simulink model "case4"  (R2024b)
settings: Solver=FixedStepAuto  StartTime=0  StopTime=1  FixedStep=1e-7  RelTol=1e-3
values from neighbouring files (symbols this model uses):
  SG_D_1_D = 0.01056    [IEEE9_case_parameters.m]    (also in case1_parameters.m; case2_parameters.m; case3_parameters.m; case4_parameters.m)
  SG_D_1_EnableSaturation = 0    [IEEE9_case_parameters.m]    (also in case1_parameters.m; case2_parameters.m; case3_parameters.m; case4_parameters.m)
  SG_D_1_f0 = 60    [IEEE9_case_parameters.m]    (also in case1_parameters.m; case2_parameters.m; case3_parameters.m; case4_parameters.m)
  SG_D_1_H = 7.5    [IEEE9_case_parameters.m]    (also in case1_parameters.m; case2_parameters.m; case3_parameters.m; case4_parameters.m)
  SG_D_1_K_A = 20    [IEEE9_case_parameters.m]    (also in case1_parameters.m; case2_parameters.m; case3_parameters.m; case4_parameters.m)
  SG_D_1_K_E = 1.000000e+1    (= 10)    [IEEE9_case_parameters.m]    (also in case1_parameters.m; case2_parameters.m; case3_parameters.m; case4_parameters.m)
  SG_D_1_K_F = 2.363    [IEEE9_case_parameters.m]    (also in case1_parameters.m; case2_parameters.m; case3_parameters.m; case4_parameters.m)
  SG_D_1_K_s = 0.5    [IEEE9_case_parameters.m]    (also in case1_parameters.m = 5; case2_parameters.m = 5; case3_parameters.m = 5; case4_parameters.m = 5)
  SG_D_1_R_a = 0.001088    [IEEE9_case_parameters.m]    (also in case1_parameters.m; case2_parameters.m; case3_parameters.m; case4_parameters.m)
  SG_D_1_S_A = 1    [IEEE9_case_parameters.m]    (also in case1_parameters.m; case2_parameters.m; case3_parameters.m; case4_parameters.m)
  SG_D_1_S_B = 0.103    [IEEE9_case_parameters.m]    (also in case1_parameters.m; case2_parameters.m; case3_parameters.m; case4_parameters.m)
  SG_D_1_S_N = 10.659857    [IEEE9_case_parameters.m]    (also in case1_parameters.m; case2_parameters.m; case3_parameters.m; case4_parameters.m)
  SG_D_1_SpeedPara = 200    [IEEE9_case_parameters.m]    (also in case1_parameters.m; case2_parameters.m; case3_parameters.m; case4_parameters.m)
  SG_D_1_T_0 = 0.720173    [IEEE9_case_parameters.m]    (also in case1_parameters.m = 0.755522; case2_parameters.m = 0.808931; case3_parameters.m = 0.869402; case4_parameters.m = 0.729316)
  SG_D_1_T_1 = 0.3    [IEEE9_case_parameters.m]    (also in case1_parameters.m; case2_parameters.m; case3_parameters.m; case4_parameters.m)
  SG_D_1_T_2 = 0.05    [IEEE9_case_parameters.m]    (also in case1_parameters.m; case2_parameters.m; case3_parameters.m; case4_parameters.m)
  SG_D_1_T_3 = 0.02    [IEEE9_case_parameters.m]    (also in case1_parameters.m; case2_parameters.m; case3_parameters.m; case4_parameters.m)
  SG_D_1_T_4 = 0.005    [IEEE9_case_parameters.m]    (also in case1_parameters.m; case2_parameters.m; case3_parameters.m; case4_parameters.m)
  SG_D_1_T_A = 0.02    [IEEE9_case_parameters.m]    (also in case1_parameters.m; case2_parameters.m; case3_parameters.m; case4_parameters.m)
  SG_D_1_T_dd = 8.000000e+0    (= 8)    [IEEE9_case_parameters.m]    (also in case1_parameters.m; case2_parameters.m; case3_parameters.m; case4_parameters.m)
  SG_D_1_T_ddd = 0.04    [IEEE9_case_parameters.m]    (also in case1_parameters.m; case2_parameters.m; case3_parameters.m; case4_parameters.m)
  SG_D_1_T_E = 0.314    [IEEE9_case_parameters.m]    (also in case1_parameters.m; case2_parameters.m; case3_parameters.m; case4_parameters.m)
  SG_D_1_T_F = 0.35    [IEEE9_case_parameters.m]    (also in case1_parameters.m; case2_parameters.m; case3_parameters.m; case4_parameters.m)
  SG_D_1_T_qd = 0.8    [IEEE9_case_parameters.m]    (also in case1_parameters.m; case2_parameters.m; case3_parameters.m; case4_parameters.m)
  SG_D_1_T_qdd = 0.02    [IEEE9_case_parameters.m]    (also in case1_parameters.m; case2_parameters.m; case3_parameters.m; case4_parameters.m)
  SG_D_1_T_speed = 0.1    [IEEE9_case_parameters.m]    (also in case1_parameters.m = 200; case2_parameters.m = 200; case3_parameters.m = 200; case4_parameters.m = 200)
  SG_D_1_T_w = 0.5    [IEEE9_case_parameters.m]    (also in case1_parameters.m; case2_parameters.m; case3_parameters.m; case4_parameters.m)
  SG_D_1_V_ref = 1.990276    [IEEE9_case_parameters.m]    (also in case1_parameters.m = 2.042296; case2_parameters.m = 2.051388; case3_parameters.m = 2.089584; case4_parameters.m = 2.01845)
  SG_D_1_w_ref = 376.991118    [IEEE9_case_parameters.m]    (also in case1_parameters.m; case2_parameters.m; case3_parameters.m; case4_parameters.m)
  SG_D_1_wb = 6.000000e+1    (= 60)    [IEEE9_case_parameters.m]    (also in case1_parameters.m; case2_parameters.m; case3_parameters.m; case4_parameters.m)
  SG_D_1_x_d = 1.9    [IEEE9_case_parameters.m]    (also in case1_parameters.m; case2_parameters.m; case3_parameters.m; case4_parameters.m)
  SG_D_1_x_dd = 0.302    [IEEE9_case_parameters.m]    (also in case1_parameters.m; case2_parameters.m; case3_parameters.m; case4_parameters.m)
  SG_D_1_x_ddd = 0.204    [IEEE9_case_parameters.m]    (also in case1_parameters.m; case2_parameters.m; case3_parameters.m; case4_parameters.m)
  SG_D_1_x_l = 0.05    [IEEE9_case_parameters.m]    (also in case1_parameters.m; case2_parameters.m; case3_parameters.m; case4_parameters.m)
  SG_D_1_x_q = 1.3    [IEEE9_case_parameters.m]    (also in case1_parameters.m; case2_parameters.m; case3_parameters.m; case4_parameters.m)
  SG_D_1_x_qd = 0.5    [IEEE9_case_parameters.m]    (also in case1_parameters.m; case2_parameters.m; case3_parameters.m; case4_parameters.m)
  SG_D_1_x_qdd = 0.3    [IEEE9_case_parameters.m]    (also in case1_parameters.m; case2_parameters.m; case3_parameters.m; case4_parameters.m)
  SG_D_2_D = 0.02    [IEEE9_case_parameters.m]    (also in case1_parameters.m; case2_parameters.m; case3_parameters.m; case4_parameters.m)
  SG_D_2_EnableSaturation = 0    [IEEE9_case_parameters.m]    (also in case1_parameters.m; case2_parameters.m; case3_parameters.m; case4_parameters.m)
  SG_D_2_f0 = 60    [IEEE9_case_parameters.m]    (also in case1_parameters.m; case2_parameters.m; case3_parameters.m; case4_parameters.m)
  SG_D_2_H = 8.000000e+0    (= 8)    [IEEE9_case_parameters.m]    (also in case1_parameters.m; case2_parameters.m; case3_parameters.m; case4_parameters.m)
  SG_D_2_K_A = 20    [IEEE9_case_parameters.m]    (also in case1_parameters.m; case2_parameters.m; case3_parameters.m; case4_parameters.m)
  SG_D_2_K_E = 1.000000e+1    (= 10)    [IEEE9_case_parameters.m]    (also in case1_parameters.m; case2_parameters.m; case3_parameters.m; case4_parameters.m)
  SG_D_2_K_F = 2.363    [IEEE9_case_parameters.m]    (also in case1_parameters.m; case2_parameters.m; case3_parameters.m; case4_parameters.m)
  SG_D_2_K_s = 0.5    [IEEE9_case_parameters.m]    (also in case1_parameters.m = 4; case2_parameters.m = 4; case3_parameters.m = 4; case4_parameters.m = 4)
  SG_D_2_R_a = 0.001088    [IEEE9_case_parameters.m]    (also in case1_parameters.m; case2_parameters.m; case3_parameters.m; case4_parameters.m)
  SG_D_2_S_A = 1    [IEEE9_case_parameters.m]    (also in case1_parameters.m; case2_parameters.m; case3_parameters.m; case4_parameters.m)
  SG_D_2_S_B = 0.103    [IEEE9_case_parameters.m]    (also in case1_parameters.m; case2_parameters.m; case3_parameters.m; case4_parameters.m)
  SG_D_2_S_N = 10.659857    [IEEE9_case_parameters.m]    (also in case1_parameters.m; case2_parameters.m; case3_parameters.m; case4_parameters.m)
  SG_D_2_SpeedPara = 200    [IEEE9_case_parameters.m]    (also in case1_parameters.m; case2_parameters.m; case3_parameters.m; case4_parameters.m)
  SG_D_2_T_0 = 1.632913    [IEEE9_case_parameters.m]    (also in case1_parameters.m = 1.632925; case2_parameters.m = 1.632915; case3_parameters.m = 1.632914; case4_parameters.m = 1.632927)
  SG_D_2_T_1 = 0.2    [IEEE9_case_parameters.m]    (also in case1_parameters.m; case2_parameters.m; case3_parameters.m; case4_parameters.m)
  SG_D_2_T_2 = 0.05    [IEEE9_case_parameters.m]    (also in case1_parameters.m; case2_parameters.m; case3_parameters.m; case4_parameters.m)
  SG_D_2_T_3 = 0.02    [IEEE9_case_parameters.m]    (also in case1_parameters.m; case2_parameters.m; case3_parameters.m; case4_parameters.m)
  SG_D_2_T_4 = 0.005    [IEEE9_case_parameters.m]    (also in case1_parameters.m; case2_parameters.m; case3_parameters.m; case4_parameters.m)
  SG_D_2_T_A = 0.02    [IEEE9_case_parameters.m]    (also in case1_parameters.m; case2_parameters.m; case3_parameters.m; case4_parameters.m)
  SG_D_2_T_dd = 7.9    [IEEE9_case_parameters.m]    (also in case1_parameters.m; case2_parameters.m; case3_parameters.m; case4_parameters.m)
  SG_D_2_T_ddd = 0.04    [IEEE9_case_parameters.m]    (also in case1_parameters.m; case2_parameters.m; case3_parameters.m; case4_parameters.m)
  SG_D_2_T_E = 0.314    [IEEE9_case_parameters.m]    (also in case1_parameters.m; case2_parameters.m; case3_parameters.m; case4_parameters.m)
  SG_D_2_T_F = 0.35    [IEEE9_case_parameters.m]    (also in case1_parameters.m; case2_parameters.m; case3_parameters.m; case4_parameters.m)
  SG_D_2_T_qd = 0.8    [IEEE9_case_parameters.m]    (also in case1_parameters.m; case2_parameters.m; case3_parameters.m; case4_parameters.m)
  SG_D_2_T_qdd = 0.015    [IEEE9_case_parameters.m]    (also in case1_parameters.m; case2_parameters.m; case3_parameters.m; case4_parameters.m)
  SG_D_2_T_speed = 0.1    [IEEE9_case_parameters.m]    (also in case1_parameters.m = 150; case2_parameters.m = 150; case3_parameters.m = 150; case4_parameters.m = 150)
  SG_D_2_T_w = 0.35    [IEEE9_case_parameters.m]    (also in case1_parameters.m; case2_parameters.m; case3_parameters.m; case4_parameters.m)
  SG_D_2_V_ref = 2.58547    [IEEE9_case_parameters.m]    (also in case1_parameters.m = 2.597896; case2_parameters.m = 2.587136; case3_parameters.m = 2.586042; case4_parameters.m = 2.599679)
  SG_D_2_w_ref = 376.991118    [IEEE9_case_parameters.m]    (also in case1_parameters.m; case2_parameters.m; case3_parameters.m; case4_parameters.m)
  SG_D_2_wb = 6.000000e+1    (= 60)    [IEEE9_case_parameters.m]    (also in case1_parameters.m; case2_parameters.m; case3_parameters.m; case4_parameters.m)
  SG_D_2_x_d = 1.8    [IEEE9_case_parameters.m]    (also in case1_parameters.m; case2_parameters.m; case3_parameters.m; case4_parameters.m)
  SG_D_2_x_dd = 0.302    [IEEE9_case_parameters.m]    (also in case1_parameters.m; case2_parameters.m; case3_parameters.m; case4_parameters.m)
  SG_D_2_x_ddd = 0.204    [IEEE9_case_parameters.m]    (also in case1_parameters.m; case2_parameters.m; case3_parameters.m; case4_parameters.m)
  SG_D_2_x_l = 0.05    [IEEE9_case_parameters.m]    (also in case1_parameters.m; case2_parameters.m; case3_parameters.m; case4_parameters.m)
  SG_D_2_x_q = 1.25    [IEEE9_case_parameters.m]    (also in case1_parameters.m; case2_parameters.m; case3_parameters.m; case4_parameters.m)
  SG_D_2_x_qd = 0.5    [IEEE9_case_parameters.m]    (also in case1_parameters.m; case2_parameters.m; case3_parameters.m; case4_parameters.m)
  SG_D_2_x_qdd = 0.3    [IEEE9_case_parameters.m]    (also in case1_parameters.m; case2_parameters.m; case3_parameters.m; case4_parameters.m)
  SG_D_3_D = 0.02    [IEEE9_case_parameters.m]    (also in case1_parameters.m; case2_parameters.m; case3_parameters.m; case4_parameters.m)
  SG_D_3_EnableSaturation = 0    [IEEE9_case_parameters.m]    (also in case1_parameters.m; case2_parameters.m; case3_parameters.m; case4_parameters.m)
  SG_D_3_f0 = 60    [IEEE9_case_parameters.m]    (also in case1_parameters.m; case2_parameters.m; case3_parameters.m; case4_parameters.m)
  SG_D_3_H = 7.7    [IEEE9_case_parameters.m]    (also in case1_parameters.m; case2_parameters.m; case3_parameters.m; case4_parameters.m)
  SG_D_3_K_A = 20    [IEEE9_case_parameters.m]    (also in case1_parameters.m; case2_parameters.m; case3_parameters.m; case4_parameters.m)
  SG_D_3_K_E = 1.000000e+1    (= 10)    [IEEE9_case_parameters.m]    (also in case1_parameters.m; case2_parameters.m; case3_parameters.m; case4_parameters.m)
  SG_D_3_K_F = 2.363    [IEEE9_case_parameters.m]    (also in case1_parameters.m; case2_parameters.m; case3_parameters.m; case4_parameters.m)
  SG_D_3_K_s = 0.2    [IEEE9_case_parameters.m]    (also in case1_parameters.m = 2; case2_parameters.m = 2; case3_parameters.m = 2; case4_parameters.m = 2)
  SG_D_3_R_a = 0.001088    [IEEE9_case_parameters.m]    (also in case1_parameters.m; case2_parameters.m; case3_parameters.m; case4_parameters.m)
  SG_D_3_S_A = 1    [IEEE9_case_parameters.m]    (also in case1_parameters.m; case2_parameters.m; case3_parameters.m; case4_parameters.m)
  SG_D_3_S_B = 0.103    [IEEE9_case_parameters.m]    (also in case1_parameters.m; case2_parameters.m; case3_parameters.m; case4_parameters.m)
  SG_D_3_S_N = 10.659857    [IEEE9_case_parameters.m]    (also in case1_parameters.m; case2_parameters.m; case3_parameters.m; case4_parameters.m)
  SG_D_3_SpeedPara = 200    [IEEE9_case_parameters.m]    (also in case1_parameters.m; case2_parameters.m; case3_parameters.m; case4_parameters.m)
  SG_D_3_T_0 = 0.850788    [IEEE9_case_parameters.m]    (also in case1_parameters.m = 0.850786; case2_parameters.m = 0.850787; case3_parameters.m; case4_parameters.m = 0.850786)
  SG_D_3_T_1 = 0.2    [IEEE9_case_parameters.m]    (also in case1_parameters.m; case2_parameters.m; case3_parameters.m; case4_parameters.m)
  SG_D_3_T_2 = 0.05    [IEEE9_case_parameters.m]    (also in case1_parameters.m; case2_parameters.m; case3_parameters.m; case4_parameters.m)
  SG_D_3_T_3 = 0.02    [IEEE9_case_parameters.m]    (also in case1_parameters.m; case2_parameters.m; case3_parameters.m; case4_parameters.m)
  SG_D_3_T_4 = 0.005    [IEEE9_case_parameters.m]    (also in case1_parameters.m; case2_parameters.m; case3_parameters.m; case4_parameters.m)
  SG_D_3_T_A = 0.02    [IEEE9_case_parameters.m]    (also in case1_parameters.m; case2_parameters.m; case3_parameters.m; case4_parameters.m)
  SG_D_3_T_dd = 8.1    [IEEE9_case_parameters.m]    (also in case1_parameters.m; case2_parameters.m; case3_parameters.m; case4_parameters.m)
  SG_D_3_T_ddd = 0.04    [IEEE9_case_parameters.m]    (also in case1_parameters.m; case2_parameters.m; case3_parameters.m; case4_parameters.m)
  SG_D_3_T_E = 0.314    [IEEE9_case_parameters.m]    (also in case1_parameters.m; case2_parameters.m; case3_parameters.m; case4_parameters.m)
  SG_D_3_T_F = 0.35    [IEEE9_case_parameters.m]    (also in case1_parameters.m; case2_parameters.m; case3_parameters.m; case4_parameters.m)
  SG_D_3_T_qd = 0.8    [IEEE9_case_parameters.m]    (also in case1_parameters.m; case2_parameters.m; case3_parameters.m; case4_parameters.m)
  SG_D_3_T_qdd = 0.015    [IEEE9_case_parameters.m]    (also in case1_parameters.m; case2_parameters.m; case3_parameters.m; case4_parameters.m)
  SG_D_3_T_speed = 0.1    [IEEE9_case_parameters.m]    (also in case1_parameters.m = 180; case2_parameters.m = 180; case3_parameters.m = 180; case4_parameters.m = 180)
  SG_D_3_T_w = 0.4    [IEEE9_case_parameters.m]    (also in case1_parameters.m; case2_parameters.m; case3_parameters.m; case4_parameters.m)
  SG_D_3_V_ref = 1.892727    [IEEE9_case_parameters.m]    (also in case1_parameters.m = 1.906439; case2_parameters.m = 1.895535; case3_parameters.m = 1.892105; case4_parameters.m = 1.906598)
  SG_D_3_w_ref = 376.991118    [IEEE9_case_parameters.m]    (also in case1_parameters.m; case2_parameters.m; case3_parameters.m; case4_parameters.m)
  SG_D_3_wb = 6.000000e+1    (= 60)    [IEEE9_case_parameters.m]    (also in case1_parameters.m; case2_parameters.m; case3_parameters.m; case4_parameters.m)
  SG_D_3_x_d = 1.85    [IEEE9_case_parameters.m]    (also in case1_parameters.m; case2_parameters.m; case3_parameters.m; case4_parameters.m)
  SG_D_3_x_dd = 0.302    [IEEE9_case_parameters.m]    (also in case1_parameters.m; case2_parameters.m; case3_parameters.m; case4_parameters.m)
  SG_D_3_x_ddd = 0.204    [IEEE9_case_parameters.m]    (also in case1_parameters.m; case2_parameters.m; case3_parameters.m; case4_parameters.m)
  SG_D_3_x_l = 0.05    [IEEE9_case_parameters.m]    (also in case1_parameters.m; case2_parameters.m; case3_parameters.m; case4_parameters.m)
  SG_D_3_x_q = 1.2    [IEEE9_case_parameters.m]    (also in case1_parameters.m; case2_parameters.m; case3_parameters.m; case4_parameters.m)
  SG_D_3_x_qd = 0.5    [IEEE9_case_parameters.m]    (also in case1_parameters.m; case2_parameters.m; case3_parameters.m; case4_parameters.m)
  SG_D_3_x_qdd = 0.3    [IEEE9_case_parameters.m]    (also in case1_parameters.m; case2_parameters.m; case3_parameters.m; case4_parameters.m)
(part 4 of 12)

== system case4/AC_1/d_vq_bus_7_block ==
  note: d_vq_bus_7 in case4
      | $2106.09563369148\,\mathrm{iq}_{\mathrm{bus},7}-376.991118430775\,\mathrm{vd}_{\mathrm{bus},7}$
      | Automatically generated on 2025-10-31 19:07:32 .
  Alge_iq_bus_7_a187d : Inport
  State_vd_bus_7_abf75 : Inport  Port=2
  Constant_2106.09563369148_e620c : Constant  Value=2106.09563369148
  Constant_376.991118430775_7228e : Constant  Value=376.991118430775
  Product_2f562 : Product
  Product_863a6 : Product
  Subtract_ba788 : Sum  Inputs=+-
  Blockout_d_vq_bus_7_f8968 : Outport
  wires:
  Constant_2106.09563369148_e620c/1 -> Product_2f562/1
  Product_863a6/1 -> Subtract_ba788/2
  Alge_iq_bus_7_a187d/1 -> Product_2f562/2
  Constant_376.991118430775_7228e/1 -> Product_863a6/1
  Subtract_ba788/1 -> Blockout_d_vq_bus_7_f8968/1
  State_vd_bus_7_abf75/1 -> Product_863a6/2
  Product_2f562/1 -> Subtract_ba788/1

== system case4/AC_1/d_vq_bus_8_block ==
  note: d_vq_bus_8 in case4
      | $1657.10381727813\,\mathrm{iq}_{\mathrm{bus},8}-376.991118430775\,\mathrm{vd}_{\mathrm{bus},8}$
      | Automatically generated on 2025-10-31 19:07:34 .
  Alge_iq_bus_8_9b29c : Inport
  State_vd_bus_8_14918 : Inport  Port=2
  Constant_1657.10381727813_3cf0f : Constant  Value=1657.10381727813
  Constant_376.991118430775_38ca6 : Constant  Value=376.991118430775
  Product_3ddfe : Product
  Product_639f3 : Product
  Subtract_26c78 : Sum  Inputs=+-
  Blockout_d_vq_bus_8_3ee0b : Outport
  wires:
  Constant_1657.10381727813_3cf0f/1 -> Product_3ddfe/1
  Constant_376.991118430775_38ca6/1 -> Product_639f3/1
  Alge_iq_bus_8_9b29c/1 -> Product_3ddfe/2
  State_vd_bus_8_14918/1 -> Product_639f3/2
  Product_3ddfe/1 -> Subtract_26c78/1
  Product_639f3/1 -> Subtract_26c78/2
  Subtract_26c78/1 -> Blockout_d_vq_bus_8_3ee0b/1

== system case4/AC_1/d_vq_bus_9_block ==
  note: d_vq_bus_9 in case4
      | $1564.27849971276\,\mathrm{iq}_{\mathrm{bus},9}-376.991118430775\,\mathrm{vd}_{\mathrm{bus},9}$
      | Automatically generated on 2025-10-31 19:07:35 .
  Alge_iq_bus_9_c8820 : Inport
  State_vd_bus_9_5e7c3 : Inport  Port=2
  Constant_1564.27849971276_69eb4 : Constant  Value=1564.27849971276
  Constant_376.991118430775_a1ef0 : Constant  Value=376.991118430775
  Product_adb94 : Product
  Product_c35c3 : Product
  Subtract_0c4fa : Sum  Inputs=+-
  Blockout_d_vq_bus_9_ae447 : Outport
  wires:
  Constant_1564.27849971276_69eb4/1 -> Product_c35c3/1
  Constant_376.991118430775_a1ef0/1 -> Product_adb94/1
  Alge_iq_bus_9_c8820/1 -> Product_c35c3/2
  State_vd_bus_9_5e7c3/1 -> Product_adb94/2
  Product_c35c3/1 -> Subtract_0c4fa/1
  Product_adb94/1 -> Subtract_0c4fa/2
  Subtract_0c4fa/1 -> Blockout_d_vq_bus_9_ae447/1

== system case4/AC_1/id_bus_1_block ==
  note: id_bus_1 in case4
      | $\mathrm{id}_{\mathrm{SG},D,1}-\mathrm{id}_{\mathrm{line},1,4}$
      | Automatically generated on 2025-10-31 19:08:04 .
  Input_id_SG_D_1_73334 : Inport
  State_id_line_1_4_ee531 : Inport  Port=2
  Subtract_490f2 : Sum  Inputs=+-
  Blockout_id_bus_1_00a24 : Outport
  wires:
  Input_id_SG_D_1_73334/1 -> Subtract_490f2/1
  State_id_line_1_4_ee531/1 -> Subtract_490f2/2
  Subtract_490f2/1 -> Blockout_id_bus_1_00a24/1

== system case4/AC_1/id_bus_2_block ==
  note: id_bus_2 in case4
      | $\mathrm{id}_{\mathrm{SG},D,2}+\mathrm{id}_{\mathrm{line},8,2}$
      | Automatically generated on 2025-10-31 19:08:07 .
  Input_id_SG_D_2_fbcda : Inport
  State_id_line_8_2_cfe5e : Inport  Port=2
  Add_11ac2 : Sum
  Blockout_id_bus_2_d0074 : Outport
  wires:
  Input_id_SG_D_2_fbcda/1 -> Add_11ac2/1
  State_id_line_8_2_cfe5e/1 -> Add_11ac2/2
  Add_11ac2/1 -> Blockout_id_bus_2_d0074/1

== system case4/AC_1/id_bus_3_block ==
  note: id_bus_3 in case4
      | $\mathrm{id}_{\mathrm{SG},D,3}-\mathrm{id}_{\mathrm{line},3,6}$
      | Automatically generated on 2025-10-31 19:08:09 .
  Input_id_SG_D_3_1ed07 : Inport
  State_id_line_3_6_05496 : Inport  Port=2
  Subtract_1ce5f : Sum  Inputs=+-
  Blockout_id_bus_3_9729d : Outport
  wires:
  Input_id_SG_D_3_1ed07/1 -> Subtract_1ce5f/1
  State_id_line_3_6_05496/1 -> Subtract_1ce5f/2
  Subtract_1ce5f/1 -> Blockout_id_bus_3_9729d/1

== system case4/AC_1/id_bus_4_block ==
  note: id_bus_4 in case4
      | $\mathrm{id}_{\mathrm{line},1,4}-\mathrm{id}_{\mathrm{line},4,5}+\mathrm{id}_{\mathrm{line},9,4}$
      | Automatically generated on 2025-10-31 19:08:10 .
  State_id_line_1_4_a86fb : Inport
  State_id_line_4_5_25293 : Inport  Port=2
  State_id_line_9_4_32915 : Inport  Port=3
  Add_ea890 : Sum
  Subtract_f741b : Sum  Inputs=+-
  Blockout_id_bus_4_42f24 : Outport
  wires:
  State_id_line_9_4_32915/1 -> Add_ea890/2
  State_id_line_1_4_a86fb/1 -> Subtract_f741b/1
  State_id_line_4_5_25293/1 -> Subtract_f741b/2
  Subtract_f741b/1 -> Add_ea890/1
  Add_ea890/1 -> Blockout_id_bus_4_42f24/1

== system case4/AC_1/id_bus_5_block ==
  note: id_bus_5 in case4
      | $\mathrm{id}_{\mathrm{line},4,5}-\mathrm{id}_{\mathrm{load},5}-\mathrm{id}_{\mathrm{line},5,6}$
      | Automatically generated on 2025-10-31 19:08:12 .
  State_id_load_5_ce210 : Inport
  State_id_line_4_5_86da7 : Inport  Port=2
  State_id_line_5_6_37460 : Inport  Port=3
  Add_495f7 : Sum
  Constant_-1_405b2 : Constant  Value=-1
  Product_41ded : Product
  Subtract_56e37 : Sum  Inputs=+-
  Blockout_id_bus_5_00d6f : Outport
  wires:
  Subtract_56e37/1 -> Blockout_id_bus_5_00d6f/1
  State_id_line_4_5_86da7/1 -> Add_495f7/2
  Constant_-1_405b2/1 -> Product_41ded/1
  Add_495f7/1 -> Subtract_56e37/1
  State_id_load_5_ce210/1 -> Product_41ded/2
  Product_41ded/1 -> Add_495f7/1
  State_id_line_5_6_37460/1 -> Subtract_56e37/2

== system case4/AC_1/id_bus_6_block ==
  note: id_bus_6 in case4
      | $\mathrm{id}_{\mathrm{line},3,6}+\mathrm{id}_{\mathrm{line},5,6}-\mathrm{id}_{\mathrm{line},6,7}$
      | Automatically generated on 2025-10-31 19:08:13 .
  State_id_line_3_6_de78e : Inport
  State_id_line_5_6_1a694 : Inport  Port=2
  State_id_line_6_7_1ddf3 : Inport  Port=3
  Add_b3029 : Sum
  Subtract_06215 : Sum  Inputs=+-
  Blockout_id_bus_6_23bdb : Outport
  wires:
  State_id_line_6_7_1ddf3/1 -> Subtract_06215/2
  State_id_line_3_6_de78e/1 -> Add_b3029/1
  State_id_line_5_6_1a694/1 -> Add_b3029/2
  Add_b3029/1 -> Subtract_06215/1
  Subtract_06215/1 -> Blockout_id_bus_6_23bdb/1

== system case4/AC_1/id_bus_7_block ==
  note: id_bus_7 in case4
      | $\mathrm{id}_{\mathrm{line},6,7}-\mathrm{id}_{\mathrm{load},7}-\mathrm{id}_{\mathrm{line},7,8}$
      | Automatically generated on 2025-10-31 19:08:14 .
  State_id_load_7_08a11 : Inport
  State_id_line_6_7_3a993 : Inport  Port=2
  State_id_line_7_8_7bb7d : Inport  Port=3
  Add_165c5 : Sum
  Constant_-1_3b2a9 : Constant  Value=-1
  Product_6f470 : Product
  Subtract_6c348 : Sum  Inputs=+-
  Blockout_id_bus_7_de2dd : Outport
  wires:
  Subtract_6c348/1 -> Blockout_id_bus_7_de2dd/1
  State_id_line_6_7_3a993/1 -> Add_165c5/2
  Constant_-1_3b2a9/1 -> Product_6f470/1
  Add_165c5/1 -> Subtract_6c348/1
  State_id_load_7_08a11/1 -> Product_6f470/2
  Product_6f470/1 -> Add_165c5/1
  State_id_line_7_8_7bb7d/1 -> Subtract_6c348/2

== system case4/AC_1/id_bus_8_block ==
  note: id_bus_8 in case4
      | $\mathrm{id}_{\mathrm{line},7,8}-\mathrm{id}_{\mathrm{line},8,2}-\mathrm{id}_{\mathrm{line},8,9}$
      | Automatically generated on 2025-10-31 19:08:16 .
  State_id_line_7_8_b4fab : Inport
  State_id_line_8_2_e242b : Inport  Port=2
  State_id_line_8_9_3adb9 : Inport  Port=3
  Subtract_0bae2 : Sum  Inputs=+-
  Subtract_32f21 : Sum  Inputs=+-
  Blockout_id_bus_8_7113f : Outport
  wires:
  State_id_line_8_9_3adb9/1 -> Subtract_32f21/2
  State_id_line_7_8_b4fab/1 -> Subtract_0bae2/1
  State_id_line_8_2_e242b/1 -> Subtract_0bae2/2
  Subtract_0bae2/1 -> Subtract_32f21/1
  Subtract_32f21/1 -> Blockout_id_bus_8_7113f/1

== system case4/AC_1/id_bus_9_block ==
  note: id_bus_9 in case4
      | $\mathrm{id}_{\mathrm{line},8,9}-\mathrm{id}_{\mathrm{load},9}-\mathrm{id}_{\mathrm{line},9,4}$
      | Automatically generated on 2025-10-31 19:08:17 .
  State_id_load_9_f6d0c : Inport
  State_id_line_8_9_502b6 : Inport  Port=2
  State_id_line_9_4_0d307 : Inport  Port=3
  Add_18cdf : Sum
  Constant_-1_14996 : Constant  Value=-1
  Product_22f20 : Product
  Subtract_385ae : Sum  Inputs=+-
  Blockout_id_bus_9_09ef3 : Outport
  wires:
  Subtract_385ae/1 -> Blockout_id_bus_9_09ef3/1
  State_id_line_8_9_502b6/1 -> Add_18cdf/2
  Constant_-1_14996/1 -> Product_22f20/1
  Add_18cdf/1 -> Subtract_385ae/1
  State_id_load_9_f6d0c/1 -> Product_22f20/2
  Product_22f20/1 -> Add_18cdf/1
  State_id_line_9_4_0d307/1 -> Subtract_385ae/2

== system case4/AC_1/iq_bus_1_block ==
  note: iq_bus_1 in case4
      | $\mathrm{iq}_{\mathrm{SG},D,1}-\mathrm{iq}_{\mathrm{line},1,4}$
      | Automatically generated on 2025-10-31 19:08:05 .
  Input_iq_SG_D_1_3d98d : Inport
  State_iq_line_1_4_d402f : Inport  Port=2
  Subtract_30e94 : Sum  Inputs=+-
  Blockout_iq_bus_1_acc76 : Outport
  wires:
  Input_iq_SG_D_1_3d98d/1 -> Subtract_30e94/1
  State_iq_line_1_4_d402f/1 -> Subtract_30e94/2
  Subtract_30e94/1 -> Blockout_iq_bus_1_acc76/1

== system case4/AC_1/iq_bus_2_block ==
  note: iq_bus_2 in case4
      | $\mathrm{iq}_{\mathrm{SG},D,2}+\mathrm{iq}_{\mathrm{line},8,2}$
      | Automatically generated on 2025-10-31 19:08:07 .
  Input_iq_SG_D_2_5cb3e : Inport
  State_iq_line_8_2_0316d : Inport  Port=2
  Add_ec71c : Sum
  Blockout_iq_bus_2_7f564 : Outport
  wires:
  Input_iq_SG_D_2_5cb3e/1 -> Add_ec71c/1
  State_iq_line_8_2_0316d/1 -> Add_ec71c/2
  Add_ec71c/1 -> Blockout_iq_bus_2_7f564/1

== system case4/AC_1/iq_bus_3_block ==
  note: iq_bus_3 in case4
      | $\mathrm{iq}_{\mathrm{SG},D,3}-\mathrm{iq}_{\mathrm{line},3,6}$
      | Automatically generated on 2025-10-31 19:08:10 .
  Input_iq_SG_D_3_132dc : Inport
  State_iq_line_3_6_0719c : Inport  Port=2
  Subtract_b190c : Sum  Inputs=+-
  Blockout_iq_bus_3_0e2bc : Outport
  wires:
  Input_iq_SG_D_3_132dc/1 -> Subtract_b190c/1
  State_iq_line_3_6_0719c/1 -> Subtract_b190c/2
  Subtract_b190c/1 -> Blockout_iq_bus_3_0e2bc/1

== system case4/AC_1/iq_bus_4_block ==
  note: iq_bus_4 in case4
      | $\mathrm{iq}_{\mathrm{line},1,4}-\mathrm{iq}_{\mathrm{line},4,5}+\mathrm{iq}_{\mathrm{line},9,4}$
      | Automatically generated on 2025-10-31 19:08:11 .
  State_iq_line_1_4_0e1d9 : Inport
  State_iq_line_4_5_08faa : Inport  Port=2
  State_iq_line_9_4_28481 : Inport  Port=3
  Add_f51e2 : Sum
  Subtract_b2dec : Sum  Inputs=+-
  Blockout_iq_bus_4_4c52a : Outport
  wires:
  State_iq_line_1_4_0e1d9/1 -> Subtract_b2dec/1
  State_iq_line_4_5_08faa/1 -> Subtract_b2dec/2
  Subtract_b2dec/1 -> Add_f51e2/1
  State_iq_line_9_4_28481/1 -> Add_f51e2/2
  Add_f51e2/1 -> Blockout_iq_bus_4_4c52a/1

== system case4/AC_1/iq_bus_5_block ==
  note: iq_bus_5 in case4
      | $\mathrm{iq}_{\mathrm{line},4,5}-\mathrm{iq}_{\mathrm{load},5}-\mathrm{iq}_{\mathrm{line},5,6}$
      | Automatically generated on 2025-10-31 19:08:12 .
  State_iq_load_5_b9fd6 : Inport
  State_iq_line_4_5_55a5a : Inport  Port=2
  State_iq_line_5_6_1a976 : Inport  Port=3
  Add_907f0 : Sum
  Constant_-1_00da9 : Constant  Value=-1
  Product_06534 : Product
  Subtract_a5efb : Sum  Inputs=+-
  Blockout_iq_bus_5_1eb56 : Outport
  wires:
  Subtract_a5efb/1 -> Blockout_iq_bus_5_1eb56/1
  State_iq_line_4_5_55a5a/1 -> Add_907f0/2
  Constant_-1_00da9/1 -> Product_06534/1
  State_iq_load_5_b9fd6/1 -> Product_06534/2
  Product_06534/1 -> Add_907f0/1
  Add_907f0/1 -> Subtract_a5efb/1
  State_iq_line_5_6_1a976/1 -> Subtract_a5efb/2

== system case4/AC_1/iq_bus_6_block ==
  note: iq_bus_6 in case4
      | $\mathrm{iq}_{\mathrm{line},3,6}+\mathrm{iq}_{\mathrm{line},5,6}-\mathrm{iq}_{\mathrm{line},6,7}$
      | Automatically generated on 2025-10-31 19:08:14 .
  State_iq_line_3_6_bd71f : Inport
  State_iq_line_5_6_2bdce : Inport  Port=2
  State_iq_line_6_7_0fdb9 : Inport  Port=3
  Add_24d65 : Sum
  Subtract_cbb99 : Sum  Inputs=+-
  Blockout_iq_bus_6_e334f : Outport
  wires:
  State_iq_line_3_6_bd71f/1 -> Add_24d65/1
  State_iq_line_5_6_2bdce/1 -> Add_24d65/2
  Add_24d65/1 -> Subtract_cbb99/1
  State_iq_line_6_7_0fdb9/1 -> Subtract_cbb99/2
  Subtract_cbb99/1 -> Blockout_iq_bus_6_e334f/1

== system case4/AC_1/iq_bus_7_block ==
  note: iq_bus_7 in case4
      | $\mathrm{iq}_{\mathrm{line},6,7}-\mathrm{iq}_{\mathrm{load},7}-\mathrm{iq}_{\mathrm{line},7,8}$
      | Automatically generated on 2025-10-31 19:08:15 .
  State_iq_load_7_41cfc : Inport
  State_iq_line_6_7_12eee : Inport  Port=2
  State_iq_line_7_8_b62c9 : Inport  Port=3
  Add_753d4 : Sum
  Constant_-1_75bee : Constant  Value=-1
  Product_0f835 : Product
  Subtract_8ae26 : Sum  Inputs=+-
  Blockout_iq_bus_7_c21f1 : Outport
  wires:
  Subtract_8ae26/1 -> Blockout_iq_bus_7_c21f1/1
  State_iq_line_6_7_12eee/1 -> Add_753d4/2
  Constant_-1_75bee/1 -> Product_0f835/1
  State_iq_load_7_41cfc/1 -> Product_0f835/2
  Product_0f835/1 -> Add_753d4/1
  Add_753d4/1 -> Subtract_8ae26/1
  State_iq_line_7_8_b62c9/1 -> Subtract_8ae26/2

== system case4/AC_1/iq_bus_8_block ==
  note: iq_bus_8 in case4
      | $\mathrm{iq}_{\mathrm{line},7,8}-\mathrm{iq}_{\mathrm{line},8,2}-\mathrm{iq}_{\mathrm{line},8,9}$
      | Automatically generated on 2025-10-31 19:08:17 .
  State_iq_line_7_8_4e039 : Inport
  State_iq_line_8_2_39c57 : Inport  Port=2
  State_iq_line_8_9_fb39e : Inport  Port=3
  Subtract_a2a05 : Sum  Inputs=+-
  Subtract_b9b34 : Sum  Inputs=+-
  Blockout_iq_bus_8_d2159 : Outport
  wires:
  State_iq_line_7_8_4e039/1 -> Subtract_a2a05/1
  State_iq_line_8_2_39c57/1 -> Subtract_a2a05/2
  Subtract_a2a05/1 -> Subtract_b9b34/1
  State_iq_line_8_9_fb39e/1 -> Subtract_b9b34/2
  Subtract_b9b34/1 -> Blockout_iq_bus_8_d2159/1

== system case4/AC_1/iq_bus_9_block ==
  note: iq_bus_9 in case4
      | $\mathrm{iq}_{\mathrm{line},8,9}-\mathrm{iq}_{\mathrm{load},9}-\mathrm{iq}_{\mathrm{line},9,4}$
      | Automatically generated on 2025-10-31 19:08:18 .
  State_iq_load_9_5d541 : Inport
  State_iq_line_8_9_a2ec0 : Inport  Port=2
  State_iq_line_9_4_ce0dd : Inport  Port=3
  Add_b1f4a : Sum
  Constant_-1_0fbd6 : Constant  Value=-1
  Product_c56aa : Product
  Subtract_2c8e3 : Sum  Inputs=+-
  Blockout_iq_bus_9_13bf1 : Outport
  wires:
  Subtract_2c8e3/1 -> Blockout_iq_bus_9_13bf1/1
  State_iq_line_8_9_a2ec0/1 -> Add_b1f4a/2
  Constant_-1_0fbd6/1 -> Product_c56aa/1
  State_iq_load_9_5d541/1 -> Product_c56aa/2
  Product_c56aa/1 -> Add_b1f4a/1
  Add_b1f4a/1 -> Subtract_2c8e3/1
  State_iq_line_9_4_ce0dd/1 -> Subtract_2c8e3/2

== system case4/AC_1/vd_bus_1_out_block ==
  note: vd_bus_1_out in case4
      | $\mathrm{vd}_{\mathrm{bus},1}$
      | Automatically generated on 2025-10-31 19:08:03 .
  State_vd_bus_1_6cc2c : Inport
  Blockout_vd_bus_1_out_8e4f7 : Outport
  wires:
  State_vd_bus_1_6cc2c/1 -> Blockout_vd_bus_1_out_8e4f7/1

== system case4/AC_1/vd_bus_2_out_block ==
  note: vd_bus_2_out in case4
      | $\mathrm{vd}_{\mathrm{bus},2}$
      | Automatically generated on 2025-10-31 19:08:05 .
  State_vd_bus_2_27286 : Inport
  Blockout_vd_bus_2_out_114e8 : Outport
  wires:
  State_vd_bus_2_27286/1 -> Blockout_vd_bus_2_out_114e8/1

== system case4/AC_1/vd_bus_3_out_block ==
  note: vd_bus_3_out in case4
      | $\mathrm{vd}_{\mathrm{bus},3}$
      | Automatically generated on 2025-10-31 19:08:08 .
  State_vd_bus_3_4cb32 : Inport
  Blockout_vd_bus_3_out_78edb : Outport
  wires:
  State_vd_bus_3_4cb32/1 -> Blockout_vd_bus_3_out_78edb/1

== system case4/AC_1/vq_bus_1_out_block ==
  note: vq_bus_1_out in case4
      | $\mathrm{vq}_{\mathrm{bus},1}$
      | Automatically generated on 2025-10-31 19:08:04 .
  State_vq_bus_1_ae207 : Inport
  Blockout_vq_bus_1_out_74281 : Outport
  wires:
  State_vq_bus_1_ae207/1 -> Blockout_vq_bus_1_out_74281/1

== system case4/AC_1/vq_bus_2_out_block ==
  note: vq_bus_2_out in case4
      | $\mathrm{vq}_{\mathrm{bus},2}$
      | Automatically generated on 2025-10-31 19:08:06 .
  State_vq_bus_2_03ca6 : Inport
  Blockout_vq_bus_2_out_4fd53 : Outport
  wires:
  State_vq_bus_2_03ca6/1 -> Blockout_vq_bus_2_out_4fd53/1

== system case4/AC_1/vq_bus_3_out_block ==
  note: vq_bus_3_out in case4
      | $\mathrm{vq}_{\mathrm{bus},3}$
      | Automatically generated on 2025-10-31 19:08:08 .
  State_vq_bus_3_4fca5 : Inport
  Blockout_vq_bus_3_out_5791b : Outport
  wires:
  State_vq_bus_3_4fca5/1 -> Blockout_vq_bus_3_out_5791b/1

== system case4/SG_D_1/T_e_SG_D_1_block ==
  note: T_e_SG_D_1 in case4
      | $-\frac{\psi _{d,\mathrm{SG},D,1}\,\left(\psi _{q,\mathrm{SG},D,1}+\frac{\psi _{\mathrm{gq},\mathrm{SG},D,1}\,\left(x_{l}-x_{\mathrm{qdd}}\right)}{x_{l}-x_{\mathrm{qd}}}+\frac{\psi _{\mathrm{kq},\mathrm{SG},D,1}\,\left(x_{\mathrm{qd}}-x_{\mathrm{qdd}}\right)}{x_{l}-x_{\mathrm{qd}}}\right)}{x_{\mathrm{qdd}}}-\frac{\psi _{q,\mathrm{SG},D,1}\,\left(\frac{\psi _{\mathrm{1d},\mathrm{SG},D,1}\,\left(x_{\mathrm{dd}}-x_{\mathrm{ddd}}\right)}{x_{\mathrm{dd}}-x_{l}}-\psi _{d,\mathrm{SG},D,1}+\frac{\psi _{\mathrm{fd},\mathrm{SG},D,1}\,\left(x_{\mathrm{ddd}}-x_{l}\right)}{x_{\mathrm{dd}}-x_{l}}\right)}{x_{\mathrm{ddd}}}$
      | Automatically generated on 2025-10-31 19:05:01 .
  State_psi_d_SG_D_1_cf38e : Inport
  State_psi_gq_SG_D_1_e3dd4 : Inport  Port=2
  State_psi_kq_SG_D_1_0d52f : Inport  Port=3
  State_psi_q_SG_D_1_3dc92 : Inport  Port=4
  State_psi_q_SG_D_1_946b5 : Inport  Port=5
  State_psi_1d_SG_D_1_7d472 : Inport  Port=6
  State_psi_d_SG_D_1_9ff9b : Inport  Port=7
  State_psi_fd_SG_D_1_4d15b : Inport  Port=8
  Add_306ef : Sum
  Add_46ba8 : Sum
  Add_5e000 : Sum
  Add_9631e : Sum
  Add_f3a9a : Sum
  Add_fb92b : Sum
  Constant_-1_4e85c : Constant  Value=-1
  Constant_-1_b14e0 : Constant  Value=-1
  Constant_-1_c8af6 : Constant  Value=-1
  Constant_-1_d4cb3 : Constant  Value=-1
  Constant_-1_fc840 : Constant  Value=-1
  Constant_x_dd_53a2f : Constant  Value=x_dd
  Constant_x_dd_880e6 : Constant  Value=x_dd
  Constant_x_dd_9ed27 : Constant  Value=x_dd
  Constant_x_ddd_1bd98 : Constant  Value=x_ddd
  Constant_x_ddd_4d371 : Constant  Value=x_ddd
  Constant_x_ddd_c0ed3 : Constant  Value=x_ddd
  Constant_x_l_09e78 : Constant  Value=x_l
  Constant_x_l_32d0b : Constant  Value=x_l
  Constant_x_l_33d64 : Constant  Value=x_l
  Constant_x_l_6c3a5 : Constant  Value=x_l
  Constant_x_l_7392b : Constant  Value=x_l
  Constant_x_l_76a89 : Constant  Value=x_l
  Constant_x_qd_05ece : Constant  Value=x_qd
  Constant_x_qd_0a332 : Constant  Value=x_qd
  Constant_x_qd_ed25e : Constant  Value=x_qd
  Constant_x_qdd_3a38b : Constant  Value=x_qdd
  Constant_x_qdd_3f6a6 : Constant  Value=x_qdd
  Constant_x_qdd_d7f23 : Constant  Value=x_qdd
  Divide_145e2 : Product  Inputs=*/
  Divide_6647b : Product  Inputs=*/
  Divide_71ee4 : Product  Inputs=*/
  Divide_c0713 : Product  Inputs=*/
  Divide_c1df9 : Product  Inputs=*/
  Divide_ce522 : Product  Inputs=*/
  Product_121d2 : Product
  Product_2afd0 : Product
  Product_3e72d : Product
  Product_400a1 : Product
  Product_65c02 : Product
  Product_6659b : Product
  Product_6700e : Product
  Product_7f5fd : Product
  Product_9f4ad : Product
  Product_c3310 : Product
  Product_fe88e : Product
  Subtract_3b173 : Sum  Inputs=+-
  Subtract_53d86 : Sum  Inputs=+-
  Subtract_b5e76 : Sum  Inputs=+-
  Subtract_b935a : Sum  Inputs=+-
  Subtract_bc289 : Sum  Inputs=+-
  Subtract_bdca8 : Sum  Inputs=+-
  Subtract_d5f91 : Sum  Inputs=+-
  Blockout_T_e_SG_D_1_a77ad : Outport
  wires:
  Product_fe88e/1 -> Divide_6647b/1
  Product_6659b/1 -> Add_f3a9a/1
  Divide_6647b/1 -> Subtract_d5f91/1
  Constant_-1_c8af6/1 -> Product_6659b/1
  Constant_x_l_76a89/1 -> Product_6659b/2
  Constant_x_qdd_d7f23/1 -> Add_f3a9a/2
  Constant_x_qd_ed25e/1 -> Subtract_53d86/1
  Constant_-1_4e85c/1 -> Product_c3310/1
  Constant_x_qdd_3f6a6/1 -> Divide_c1df9/2
  Constant_x_qdd_3a38b/1 -> Subtract_53d86/2
  State_psi_q_SG_D_1_946b5/1 -> Product_2afd0/1
  Constant_x_dd_53a2f/1 -> Subtract_b5e76/1
  Constant_x_l_33d64/1 -> Product_c3310/2
  Subtract_b5e76/1 -> Product_121d2/2
  Constant_-1_d4cb3/1 -> Product_400a1/1
  Constant_x_l_09e78/1 -> Product_400a1/2
  Subtract_bdca8/1 -> Product_2afd0/2
  State_psi_q_SG_D_1_3dc92/1 -> Add_9631e/2
  Constant_-1_b14e0/1 -> Product_6700e/1
  State_psi_1d_SG_D_1_7d472/1 -> Product_6700e/2
  Constant_x_ddd_1bd98/1 -> Subtract_b5e76/2
  State_psi_gq_SG_D_1_e3dd4/1 -> Product_fe88e/1
  Add_f3a9a/1 -> Product_fe88e/2
  Product_c3310/1 -> Add_306ef/1
  Product_3e72d/1 -> Product_9f4ad/1
  Constant_x_qd_05ece/1 -> Add_306ef/2
  Product_121d2/1 -> Divide_c0713/1
  State_psi_kq_SG_D_1_0d52f/1 -> Product_7f5fd/1
  Add_306ef/1 -> Divide_6647b/2
  Subtract_53d86/1 -> Product_7f5fd/2
  Product_400a1/1 -> Add_fb92b/1
  Constant_x_qd_0a332/1 -> Add_fb92b/2
  Product_7f5fd/1 -> Divide_145e2/1
  Product_6700e/1 -> Product_121d2/1
  Constant_x_dd_9ed27/1 -> Subtract_b935a/1
  Constant_x_l_6c3a5/1 -> Subtract_b935a/2
  Constant_x_ddd_c0ed3/1 -> Subtract_3b173/1
  Product_2afd0/1 -> Divide_ce522/1
  Constant_x_l_32d0b/1 -> Subtract_3b173/2
  Divide_c1df9/1 -> Add_5e000/1
  Product_9f4ad/1 -> Divide_c1df9/1
  Add_fb92b/1 -> Divide_145e2/2
  Subtract_d5f91/1 -> Add_9631e/1
  Divide_145e2/1 -> Subtract_d5f91/2
  Subtract_b935a/1 -> Divide_c0713/2
  State_psi_fd_SG_D_1_4d15b/1 -> Product_65c02/1
  Constant_x_ddd_4d371/1 -> Divide_ce522/2
  Subtract_3b173/1 -> Product_65c02/2
  Constant_x_dd_880e6/1 -> Subtract_bc289/1
  Constant_x_l_7392b/1 -> Subtract_bc289/2
  Divide_c0713/1 -> Add_46ba8/1
  Add_46ba8/1 -> Subtract_bdca8/1
  State_psi_d_SG_D_1_9ff9b/1 -> Add_46ba8/2
  Product_65c02/1 -> Divide_71ee4/1
  Subtract_bc289/1 -> Divide_71ee4/2
  Constant_-1_fc840/1 -> Product_3e72d/1
  State_psi_d_SG_D_1_cf38e/1 -> Product_3e72d/2
  Divide_71ee4/1 -> Subtract_bdca8/2
  Add_9631e/1 -> Product_9f4ad/2
  Divide_ce522/1 -> Add_5e000/2
  Add_5e000/1 -> Blockout_T_e_SG_D_1_a77ad/1

== system case4/SG_D_1/d_E_fd_SG_D_1_block ==
  note: d_E_fd_SG_D_1 in case4
      | $\frac{V_{f,\mathrm{SG},D,1}-E_{\mathrm{fd},\mathrm{SG},D,1}\,K_{E}}{T_{E}}$
      | Automatically generated on 2025-10-31 19:04:45 .
  State_E_fd_SG_D_1_c0e19 : Inport
  State_V_f_SG_D_1_5ae7d : Inport  Port=2
  Add_3e585 : Sum
  Constant_-1_a976e : Constant  Value=-1
  Constant_K_E_900c0 : Constant  Value=K_E
  Constant_T_E_1d5d9 : Constant  Value=T_E
  Divide_84a20 : Product  Inputs=*/
  Product_0b372 : Product
  Product_e9582 : Product
  Blockout_d_E_fd_SG_D_1_51614 : Outport
  wires:
  Add_3e585/1 -> Divide_84a20/1
  Constant_-1_a976e/1 -> Product_0b372/1
  State_E_fd_SG_D_1_c0e19/1 -> Product_0b372/2
  Product_0b372/1 -> Product_e9582/1
  Constant_K_E_900c0/1 -> Product_e9582/2
  Product_e9582/1 -> Add_3e585/1
  Constant_T_E_1d5d9/1 -> Divide_84a20/2
  State_V_f_SG_D_1_5ae7d/1 -> Add_3e585/2
  Divide_84a20/1 -> Blockout_d_E_fd_SG_D_1_51614/1

== system case4/SG_D_1/d_Px_1_SG_D_1_block ==
  note: d_Px_1_SG_D_1 in case4
      | $\frac{w_{\mathrm{SG},D,1}-2\,\pi \,f_{0}}{T_{w}}-\frac{\mathrm{Px}_{1,\mathrm{SG},D,1}}{T_{w}}$
      | Automatically generated on 2025-10-31 19:04:46 .
  State_Px_1_SG_D_1_9d70a : Inport
  State_w_SG_D_1_192b2 : Inport  Port=2
  Add_70a3f : Sum
  Add_db824 : Sum
  Constant_-1_dc627 : Constant  Value=-1
  Constant_-2.0_90b9d : Constant  Value=-2.0
  Constant_T_w_a4e54 : Constant  Value=T_w
  Constant_T_w_c97f2 : Constant  Value=T_w
  Constant_f0_9970f : Constant  Value=f0
  Constant_pi_efdfb : Constant  Value=pi
  Divide_0d4b3 : Product  Inputs=*/
  Divide_5c609 : Product  Inputs=*/
  Product_00ba5 : Product
  Product_43a0d : Product
  Product_69ec1 : Product
  Blockout_d_Px_1_SG_D_1_c0100 : Outport
  wires:
  Add_70a3f/1 -> Blockout_d_Px_1_SG_D_1_c0100/1
  Constant_-2.0_90b9d/1 -> Product_69ec1/1
  Product_00ba5/1 -> Divide_0d4b3/1
  State_w_SG_D_1_192b2/1 -> Add_db824/2
  Constant_-1_dc627/1 -> Product_00ba5/1
  Constant_f0_9970f/1 -> Product_43a0d/2
  Constant_pi_efdfb/1 -> Product_69ec1/2
  Product_43a0d/1 -> Add_db824/1
  Product_69ec1/1 -> Product_43a0d/1
  State_Px_1_SG_D_1_9d70a/1 -> Product_00ba5/2
  Constant_T_w_c97f2/1 -> Divide_0d4b3/2
  Add_db824/1 -> Divide_5c609/1
  Constant_T_w_a4e54/1 -> Divide_5c609/2
  Divide_0d4b3/1 -> Add_70a3f/1
  Divide_5c609/1 -> Add_70a3f/2

== system case4/SG_D_1/d_Px_2_SG_D_1_block ==
  note: d_Px_2_SG_D_1 in case4
      | $\frac{\mathrm{Px}_{1,\mathrm{SG},D,1}-T_{2}\,\left(\frac{\mathrm{Px}_{1,\mathrm{SG},D,1}}{T_{w}}-\frac{w_{\mathrm{SG},D,1}-2\,\pi \,f_{0}}{T_{w}}\right)}{T_{1}}-\frac{\mathrm{Px}_{2,\mathrm{SG},D,1}}{T_{1}}$
      | Automatically generated on 2025-10-31 19:04:48 .
  State_Px_2_SG_D_1_e9b00 : Inport
  State_Px_1_SG_D_1_e74a6 : Inport  Port=2
  State_Px_1_SG_D_1_52394 : Inport  Port=3
  State_w_SG_D_1_8e384 : Inport  Port=4
  Add_189e0 : Sum
  Add_4e933 : Sum
  Add_7bdd4 : Sum
  Add_a4feb : Sum
  Constant_-1_35482 : Constant  Value=-1
  Constant_-1_50b8d : Constant  Value=-1
  Constant_-2.0_ae4ae : Constant  Value=-2.0
  Constant_T_1_a33e1 : Constant  Value=T_1
  Constant_T_1_f077e : Constant  Value=T_1
  Constant_T_2_a5da5 : Constant  Value=T_2
  Constant_T_w_53d89 : Constant  Value=T_w
  Constant_T_w_6f1d8 : Constant  Value=T_w
  Constant_f0_6c096 : Constant  Value=f0
  Constant_pi_2baca : Constant  Value=pi
  Divide_5b1f0 : Product  Inputs=*/
  Divide_a05d9 : Product  Inputs=*/
  Divide_c788c : Product  Inputs=*/
  Divide_e8244 : Product  Inputs=*/
  Product_10ef5 : Product
  Product_6f8c2 : Product
  Product_77838 : Product
  Product_857ef : Product
  Product_a8a51 : Product
  Blockout_d_Px_2_SG_D_1_bfa82 : Outport
  wires:
  Constant_-2.0_ae4ae/1 -> Product_6f8c2/1
  State_w_SG_D_1_8e384/1 -> Add_4e933/2
  Constant_f0_6c096/1 -> Product_857ef/2
  Constant_pi_2baca/1 -> Product_6f8c2/2
  Add_a4feb/1 -> Product_10ef5/2
  Product_857ef/1 -> Add_4e933/1
  Divide_e8244/1 -> Add_a4feb/1
  Product_6f8c2/1 -> Product_857ef/1
  Constant_T_w_53d89/1 -> Divide_e8244/2
  Constant_-1_35482/1 -> Product_77838/1
  State_Px_1_SG_D_1_52394/1 -> Product_77838/2
  Divide_a05d9/1 -> Add_189e0/1
  Product_77838/1 -> Divide_e8244/1
  Add_4e933/1 -> Divide_c788c/1
  Constant_T_w_6f1d8/1 -> Divide_c788c/2
  Divide_c788c/1 -> Add_a4feb/2
  Constant_T_2_a5da5/1 -> Product_10ef5/1
  Constant_-1_50b8d/1 -> Product_a8a51/1
  State_Px_2_SG_D_1_e9b00/1 -> Product_a8a51/2
  State_Px_1_SG_D_1_e74a6/1 -> Add_7bdd4/1
  Product_10ef5/1 -> Add_7bdd4/2
  Add_7bdd4/1 -> Divide_5b1f0/1
  Product_a8a51/1 -> Divide_a05d9/1
  Constant_T_1_f077e/1 -> Divide_a05d9/2
  Constant_T_1_a33e1/1 -> Divide_5b1f0/2
  Divide_5b1f0/1 -> Add_189e0/2
  Add_189e0/1 -> Blockout_d_Px_2_SG_D_1_bfa82/1

== system case4/SG_D_1/d_Px_3_SG_D_1_block ==
  note: d_Px_3_SG_D_1 in case4
      | $\frac{\mathrm{Px}_{2,\mathrm{SG},D,1}+T_{4}\,\left(\frac{\mathrm{Px}_{1,\mathrm{SG},D,1}-T_{2}\,\left(\frac{\mathrm{Px}_{1,\mathrm{SG},D,1}}{T_{w}}-\frac{w_{\mathrm{SG},D,1}-2\,\pi \,f_{0}}{T_{w}}\right)}{T_{1}}-\frac{\mathrm{Px}_{2,\mathrm{SG},D,1}}{T_{1}}\right)}{T_{3}}-\frac{\mathrm{Px}_{3,\mathrm{SG},D,1}}{T_{3}}$
      | Automatically generated on 2025-10-31 19:04:50 .
  State_Px_3_SG_D_1_45f45 : Inport
  State_Px_2_SG_D_1_89bd0 : Inport  Port=2
  State_Px_2_SG_D_1_28cf3 : Inport  Port=3
  State_Px_1_SG_D_1_408f6 : Inport  Port=4
  State_Px_1_SG_D_1_97917 : Inport  Port=5
  State_w_SG_D_1_924cf : Inport  Port=6
  Add_4514c : Sum
  Add_5705c : Sum
  Add_59c7b : Sum
  Add_5d6ba : Sum
  Add_a4622 : Sum
  Add_d8fea : Sum
  Constant_-1_5eb31 : Constant  Value=-1
  Constant_-1_86fa4 : Constant  Value=-1
  Constant_-1_bf025 : Constant  Value=-1
  Constant_-2.0_962c6 : Constant  Value=-2.0
  Constant_T_1_489fa : Constant  Value=T_1
  Constant_T_1_735e4 : Constant  Value=T_1
  Constant_T_2_8d4e9 : Constant  Value=T_2
  Constant_T_3_72389 : Constant  Value=T_3
  Constant_T_3_98b8a : Constant  Value=T_3
  Constant_T_4_33200 : Constant  Value=T_4
  Constant_T_w_130e7 : Constant  Value=T_w
  Constant_T_w_230da : Constant  Value=T_w
  Constant_f0_8da91 : Constant  Value=f0
  Constant_pi_79eaf : Constant  Value=pi
  Divide_78625 : Product  Inputs=*/
  Divide_7f2b1 : Product  Inputs=*/
  Divide_c9c6a : Product  Inputs=*/
  Divide_c9e00 : Product  Inputs=*/
  Divide_ec55d : Product  Inputs=*/
  Divide_f800f : Product  Inputs=*/
  Product_337db : Product
  Product_3c72b : Product
  Product_7ea70 : Product
  Product_a2331 : Product
  Product_c74e0 : Product
  Product_faba2 : Product
  Product_fe5d5 : Product
  Blockout_d_Px_3_SG_D_1_80a90 : Outport
  wires:
  Constant_T_w_130e7/1 -> Divide_7f2b1/2
  Constant_-1_86fa4/1 -> Product_c74e0/1
  Add_5d6ba/1 -> Blockout_d_Px_3_SG_D_1_80a90/1
  Constant_-2.0_962c6/1 -> Product_3c72b/1
  State_w_SG_D_1_924cf/1 -> Add_d8fea/2
  Constant_f0_8da91/1 -> Product_faba2/2
  State_Px_1_SG_D_1_97917/1 -> Product_c74e0/2
  Constant_pi_79eaf/1 -> Product_3c72b/2
  Product_faba2/1 -> Add_d8fea/1
  Product_3c72b/1 -> Product_faba2/1
  Product_c74e0/1 -> Divide_7f2b1/1
  Divide_78625/1 -> Add_5d6ba/1
  Constant_T_3_72389/1 -> Divide_c9c6a/2
  Add_d8fea/1 -> Divide_ec55d/1
  Constant_T_w_230da/1 -> Divide_ec55d/2
  Divide_7f2b1/1 -> Add_59c7b/1
  Divide_ec55d/1 -> Add_59c7b/2
  Constant_-1_5eb31/1 -> Product_fe5d5/1
  Constant_T_2_8d4e9/1 -> Product_a2331/1
  Add_59c7b/1 -> Product_a2331/2
  Constant_-1_bf025/1 -> Product_337db/1
  Divide_c9c6a/1 -> Add_5d6ba/2
  Constant_T_3_98b8a/1 -> Divide_78625/2
  State_Px_2_SG_D_1_28cf3/1 -> Product_337db/2
  State_Px_1_SG_D_1_408f6/1 -> Add_4514c/1
  Divide_c9e00/1 -> Add_5705c/1
  Product_a2331/1 -> Add_4514c/2
  Product_337db/1 -> Divide_c9e00/1
  Product_fe5d5/1 -> Divide_78625/1
  Constant_T_1_489fa/1 -> Divide_c9e00/2
  Add_4514c/1 -> Divide_f800f/1
  Constant_T_1_735e4/1 -> Divide_f800f/2
  Divide_f800f/1 -> Add_5705c/2
  Constant_T_4_33200/1 -> Product_7ea70/1
  Add_5705c/1 -> Product_7ea70/2
  State_Px_3_SG_D_1_45f45/1 -> Product_fe5d5/2
  State_Px_2_SG_D_1_89bd0/1 -> Add_a4622/1
  Product_7ea70/1 -> Add_a4622/2
  Add_a4622/1 -> Divide_c9c6a/1

== system case4/SG_D_1/d_R_f_SG_D_1_block ==
  note: d_R_f_SG_D_1 in case4
      | $-\frac{R_{f,\mathrm{SG},D,1}-\frac{E_{\mathrm{fd},\mathrm{SG},D,1}\,K_{F}}{T_{F}}}{T_{F}}$
      | Automatically generated on 2025-10-31 19:04:45 .
  State_E_fd_SG_D_1_a2a74 : Inport
  State_R_f_SG_D_1_ef266 : Inport  Port=2
  Constant_K_F_54ac1 : Constant  Value=K_F
  Constant_T_F_4f145 : Constant  Value=T_F
  Constant_T_F_95b8b : Constant  Value=T_F
  Divide_68c6e : Product  Inputs=*/
  Divide_9b49b : Product  Inputs=*/
  Product_a47be : Product
  Subtract_20a5c : Sum  Inputs=+-
  Blockout_d_R_f_SG_D_1_b6ceb : Outport
  wires:
  Constant_K_F_54ac1/1 -> Product_a47be/2
  Product_a47be/1 -> Divide_68c6e/1
  State_E_fd_SG_D_1_a2a74/1 -> Product_a47be/1
  State_R_f_SG_D_1_ef266/1 -> Subtract_20a5c/2
  Constant_T_F_95b8b/1 -> Divide_68c6e/2
  Divide_68c6e/1 -> Subtract_20a5c/1
  Divide_9b49b/1 -> Blockout_d_R_f_SG_D_1_b6ceb/1
  Subtract_20a5c/1 -> Divide_9b49b/1
  Constant_T_F_4f145/1 -> Divide_9b49b/2

== system case4/SG_D_1/d_T_m_SG_D_1_block ==
  note: d_T_m_SG_D_1 in case4
      | $-\frac{T_{m,\mathrm{SG},D,1}-T_{0}+\frac{\mathrm{SpeedPara}\,\left(w_{\mathrm{SG},D,1}-w_{\mathrm{ref}}\right)}{2\,f_{0}\,\pi }}{T_{\mathrm{speed}}}$
      | Automatically generated on 2025-10-31 19:04:35 .
  State_w_SG_D_1_428b2 : Inport
  State_T_m_SG_D_1_d0a69 : Inport  Port=2
  Add_6f4db : Sum
  Add_e9767 : Sum
  Constant_-1_94fda : Constant  Value=-1
  Constant_2.0_d80c7 : Constant  Value=2.0
  Constant_SpeedPara_69a67 : Constant  Value=SpeedPara
  Constant_T_0_79ec2 : Constant  Value=T_0
  Constant_T_speed_6773e : Constant  Value=T_speed
  Constant_f0_eb1a2 : Constant  Value=f0
  Constant_pi_fc646 : Constant  Value=pi
  Constant_w_ref_57324 : Constant  Value=w_ref
  Divide_11c44 : Product  Inputs=*/
  Divide_b6be8 : Product  Inputs=*/
  Product_1f042 : Product
  Product_6f10a : Product
  Product_81f5c : Product
  Product_f8754 : Product
  Subtract_d3778 : Sum  Inputs=+-
  Blockout_d_T_m_SG_D_1_af57e : Outport
  wires:
  Constant_-1_94fda/1 -> Product_f8754/1
  Constant_w_ref_57324/1 -> Add_6f4db/2
  State_w_SG_D_1_428b2/1 -> Product_f8754/2
  Add_e9767/1 -> Subtract_d3778/1
  Add_6f4db/1 -> Product_6f10a/2
  Product_f8754/1 -> Add_6f4db/1
  Constant_2.0_d80c7/1 -> Product_1f042/1
  Constant_pi_fc646/1 -> Product_1f042/2
  Constant_SpeedPara_69a67/1 -> Product_6f10a/1
  Product_1f042/1 -> Product_81f5c/1
  Constant_f0_eb1a2/1 -> Product_81f5c/2
  Constant_T_speed_6773e/1 -> Divide_11c44/2
  Product_6f10a/1 -> Divide_b6be8/1
  Product_81f5c/1 -> Divide_b6be8/2
  Divide_b6be8/1 -> Add_e9767/1
  Constant_T_0_79ec2/1 -> Add_e9767/2
  State_T_m_SG_D_1_d0a69/1 -> Subtract_d3778/2
  Subtract_d3778/1 -> Divide_11c44/1
  Divide_11c44/1 -> Blockout_d_T_m_SG_D_1_af57e/1
